simulink subsystem "Environment"  (R2021b)
settings: Solver=VariableStepAuto  StartTime=0.0  StopTime=10.0  RelTol=1e-3
undefined symbols (not defined in the file): env, spacecraft
settings Model: Creator=DELL  LastModifiedBy=DELL

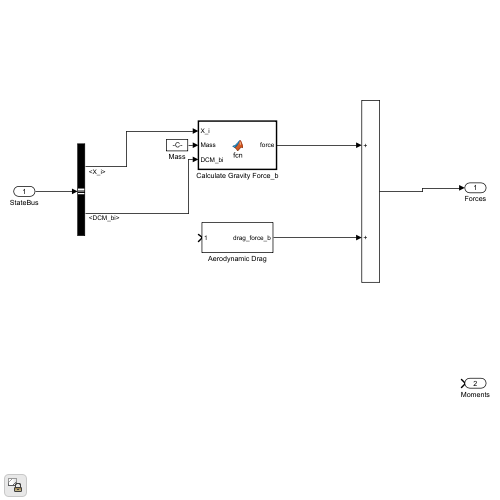
[thumbnail: Simulink's stored preview of the top-level diagram]
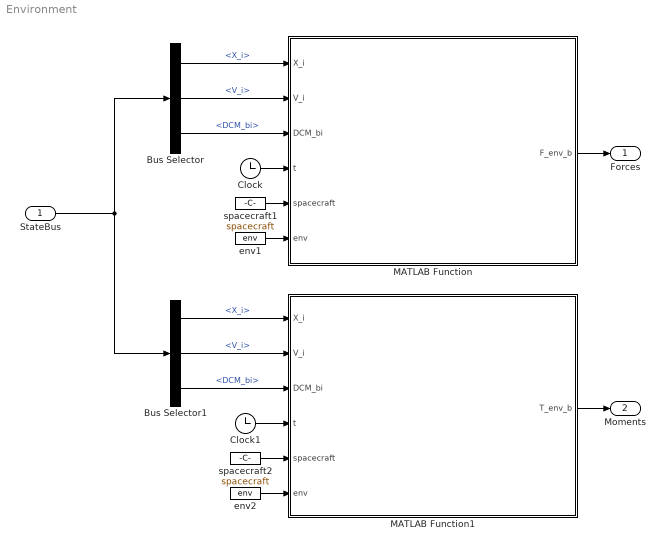
== system Environment ==
  StateBus : Inport
  Bus Selector : BusSelector  OutputSignals=X_i,V_i,DCM_bi
  Bus Selector1 : BusSelector  OutputSignals=X_i,V_i,DCM_bi
  Clock : Clock
  Clock1 : Clock
  MATLAB Function : MATLAB Function  TreatAsAtomicUnit=on
  MATLAB Function1 : MATLAB Function  TreatAsAtomicUnit=on
  env1 : Constant  Value=env  OutDataTypeStr=Bus: EnvBus
  env2 : Constant  Value=env  OutDataTypeStr=Bus: EnvBus
  spacecraft1 : Constant  Value=spacecraft  OutDataTypeStr=Bus: SpacecraftBus
  spacecraft2 : Constant  Value=spacecraft  OutDataTypeStr=Bus: SpacecraftBus
  Forces : Outport
  Moments : Outport  Port=2
  wires:
  StateBus/1 -> Bus Selector/1, Bus Selector1/1
  MATLAB Function/1(F_env_b) -> Forces/1
  MATLAB Function1/1(T_env_b) -> Moments/1
  Bus Selector/1 -> MATLAB Function/1(X_i)  "<X_i>"
  Bus Selector1/1 -> MATLAB Function1/1(X_i)  "<X_i>"
  Bus Selector/3 -> MATLAB Function/3(DCM_bi)  "<DCM_bi>"
  Bus Selector1/3 -> MATLAB Function1/3(DCM_bi)  "<DCM_bi>"
  spacecraft2/1 -> MATLAB Function1/5(spacecraft)
  env2/1 -> MATLAB Function1/6(env)
  spacecraft1/1 -> MATLAB Function/5(spacecraft)
  env1/1 -> MATLAB Function/6(env)
  Bus Selector/2 -> MATLAB Function/2(V_i)  "<V_i>"
  Bus Selector1/2 -> MATLAB Function1/2(V_i)  "<V_i>"
  Clock/1 -> MATLAB Function/4(t)
  Clock1/1 -> MATLAB Function1/4(t)

== matlab function Environment/MATLAB Function1 ==
  data: X_i input; T_env_b output; V_i input; DCM_bi input; t input; spacecraft input; env input
function T_env_b = calc_env_torques_b(X_i, V_i, DCM_bi, t, spacecraft, env)
sunVector_i = calc_sun_vector_i(t, env);
B_i = calc_magnetic_field_i(X_i, env);
T_gg_b = calc_gravity_gradient_torque_b(X_i, DCM_bi, spacecraft.inertiaKgM2, env);
T_mag_b = calc_magnetic_torque_b(B_i, DCM_bi, spacecraft.residualDipoleAm2);
T_srp_b = calc_solar_pressure_torque_b(sunVector_i, DCM_bi, spacecraft, env);
T_drag_b = calc_aerodynamic_torque_b(X_i, V_i, DCM_bi, spacecraft, env);

T_env_b = T_gg_b + T_mag_b + T_srp_b + T_drag_b;
end

== matlab function Environment/MATLAB Function ==
  data: X_i input; F_env_b output; V_i input; DCM_bi input; t input; spacecraft input; env input
function F_env_b = calc_env_forces_b(X_i, V_i, DCM_bi, t, spacecraft, env)
sunVector_i = calc_sun_vector_i(t, env);
F_gravity_b = calc_gravity_b(X_i, spacecraft.massKg, DCM_bi);
F_drag_b = calc_atmospheric_drag_b(X_i, V_i, DCM_bi, spacecraft, env);
F_srp_b = calc_solar_radiation_pressure_b(sunVector_i, DCM_bi, spacecraft, env);

F_env_b = F_gravity_b + F_drag_b + F_srp_b;
end
